simulink model "hw4_2"  (R2019a)
settings: Solver=VariableStepAuto  StartTime=0.0  StopTime=100  RelTol=1e-3
values from neighbouring files (symbols this model uses):
  EM_RPM = [0 1000 2000 3000 4000 5000 5300 6000 7000 8000 8500 9000 ... (24 elements, 1x24)]    [Electric_Motor_Data.mat]
  EM_torque_Nm = [260 260 260 260 260 260 260 260 260 260 260 246 ... (24 elements, 24x1)]    [Electric_Motor_Data.mat]
settings Model: Creator=kzhai  LastModifiedBy=kzhai

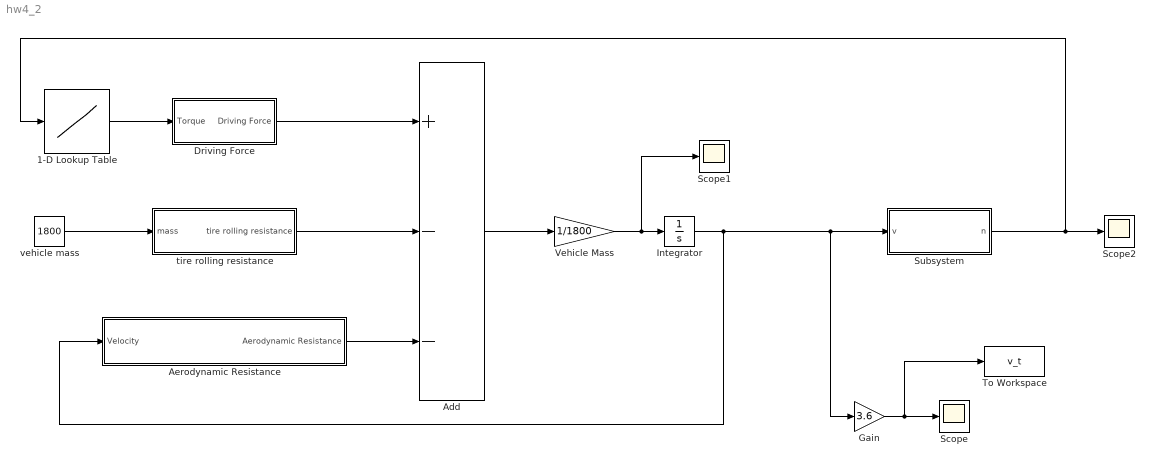
== system hw4_2 ==
  1-D Lookup Table : Lookup_n-D  NumberOfTableDimensions=1  BreakpointsForDimension1=EM_RPM  Table=EM_torque_Nm  InternalRulePriority=Speed  RndMeth=Simplest  InputSameDT=on
  Add : Sum  Inputs=+--
  "Aerodynamic Resistance " : Subsystem
  Driving Force : Subsystem
  Gain : Gain  Gain=3.6
  Integrator : Integrator
  Scope : Scope
  Scope1 : Scope
  Scope2 : Scope
  Subsystem : Subsystem
  To Workspace : ToWorkspace  VariableName=v_t  SampleTime=-1
  Vehicle Mass : Gain  Gain=1/1800
  tire rolling resistance : Subsystem
  vehicle mass : Constant  Value=1800
  wires:
  tire rolling resistance/1(tire rolling resistance) -> Add/2
  Driving Force/1(Driving Force) -> Add/1
  "Aerodynamic Resistance "/1(Aerodynamic Resistance) -> Add/3
  1-D Lookup Table/1 -> Driving Force/1(Torque)
  Add/1 -> Vehicle Mass/1
  Vehicle Mass/1 -> Scope1/1, Integrator/1
  Subsystem/1(n) -> 1-D Lookup Table/1, Scope2/1
  vehicle mass/1 -> tire rolling resistance/1(mass)
  Integrator/1 -> Gain/1, Subsystem/1(v), "Aerodynamic Resistance "/1(Velocity)
  Gain/1 -> To Workspace/1, Scope/1

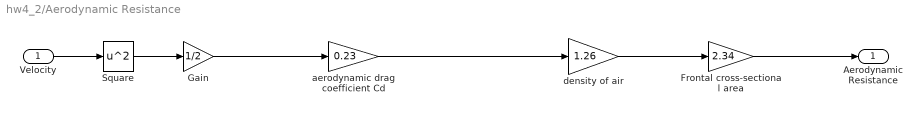
== system hw4_2/Aerodynamic Resistance  ==
  Velocity : Inport
  Frontal cross-sectional area : Gain  Gain=2.34
  Gain : Gain  Gain=1/2
  Square : Math  Operator=square  SaturateOnIntegerOverflow=on
  aerodynamic drag coefficient Cd : Gain  Gain=0.23
  density of air : Gain  Gain=1.26
  Aerodynamic Resistance : Outport
  wires:
  Frontal cross-sectional area/1 -> Aerodynamic Resistance/1
  Gain/1 -> aerodynamic drag coefficient Cd/1
  density of air/1 -> Frontal cross-sectional area/1
  Velocity/1 -> Square/1
  Square/1 -> Gain/1
  aerodynamic drag coefficient Cd/1 -> density of air/1

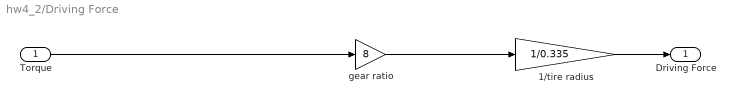
== system hw4_2/Driving Force ==
  Torque : Inport
  1/tire radius : Gain  Gain=1/0.335
  gear ratio : Gain  Gain=8
  Driving Force : Outport
  wires:
  1/tire radius/1 -> Driving Force/1
  Torque/1 -> gear ratio/1
  gear ratio/1 -> 1/tire radius/1

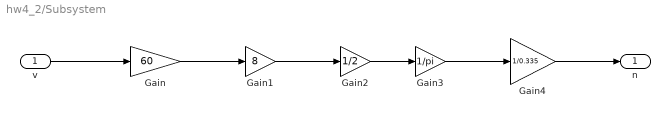
== system hw4_2/Subsystem ==
  v : Inport
  Gain : Gain  Gain=60
  Gain1 : Gain  Gain=8
  Gain2 : Gain  Gain=1/2
  Gain3 : Gain  Gain=1/pi
  Gain4 : Gain  Gain=1/0.335
  n : Outport
  wires:
  Gain/1 -> Gain1/1
  Gain1/1 -> Gain2/1
  Gain2/1 -> Gain3/1
  Gain3/1 -> Gain4/1
  v/1 -> Gain/1
  Gain4/1 -> n/1

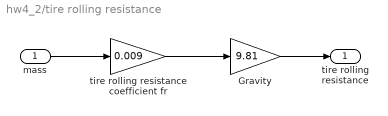
== system hw4_2/tire rolling resistance ==
  mass : Inport
  Gravity : Gain  Gain=9.81
  tire rolling resistance coefficient fr : Gain  Gain=0.009
  tire rolling resistance : Outport
  wires:
  tire rolling resistance coefficient fr/1 -> Gravity/1
  Gravity/1 -> tire rolling resistance/1
  mass/1 -> tire rolling resistance coefficient fr/1
